simulink model "Power_System_Analysis_Protection"  (R2024b)
settings: Solver=VariableStepAuto  StartTime=0.0  StopTime=0.1  RelTol=1e-3
libraries: simulink x1, spsGroundLib x1, eePowerMeasurement x1, spsRMSLib x1, spsThreePhaseProgrammableVoltageSourceLib x1, spsThreePhaseSeriesRLCLoadLib x1, spsThreePhaseTransformerTwoWindingsLib x1, spsThreePhaseVIMeasurementLib x1, spsThreePhaseBreakerLib x1, spsThreePhaseFaultLib x1, spspowerguiLib x1
settings Model: Creator=Masoom Ali  LastModifiedBy=Masoom Ali

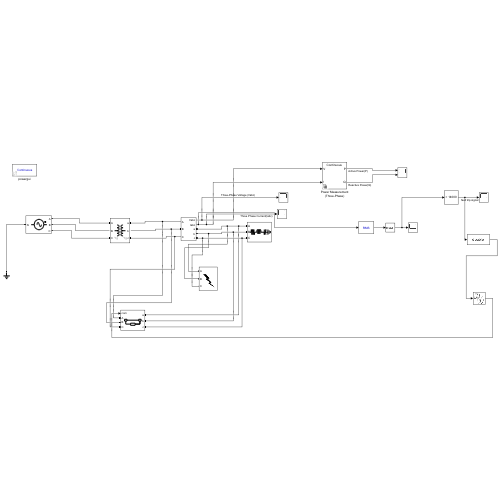
[thumbnail: Simulink's stored preview of the top-level diagram]
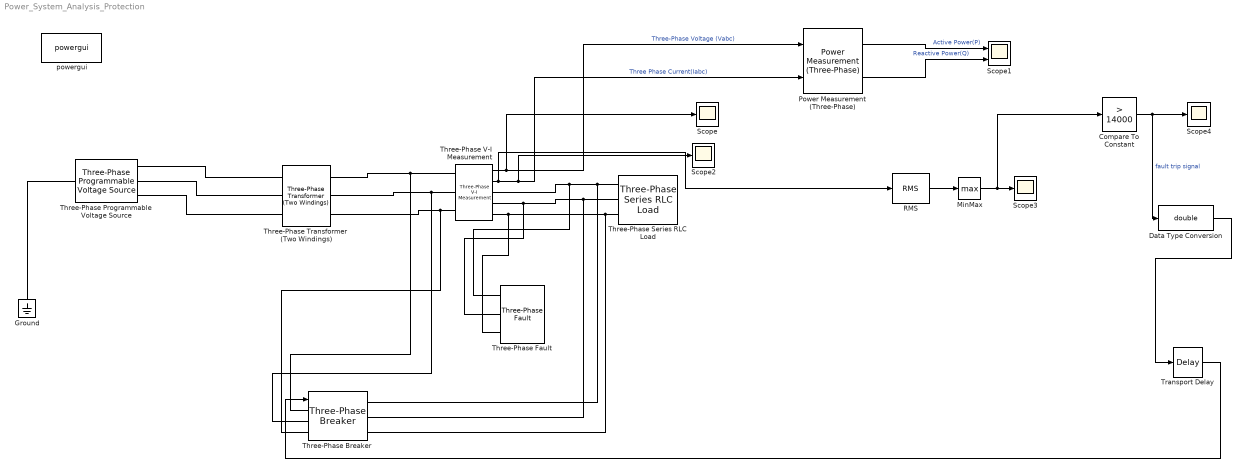
== system Power_System_Analysis_Protection ==
  Compare To Constant : simulink/Logic and Bit Operations/Compare To Constant  relop=>  const=14000  OutDataTypeStr=uint8
  Data Type Conversion : DataTypeConversion  OutDataTypeStr=double  SaturateOnIntegerOverflow=off  RndMeth=Floor
  Ground : spsGroundLib/Ground  LConnTagsString=a
  MinMax : MinMax  Function=max
  Power Measurement (Three-Phase) : eePowerMeasurement/Power Measurement (Three-Phase)  LabelModeActiveChoice=Continuous  F=50  K=1  Seq=Positive  Ts=0
  RMS : spsRMSLib/RMS  TrueRMS=on  Freq=50  RMSInit=120  Ts=0
  Scope{,2..4} (4 alike) : Scope
  Scope1 : Scope  NumInputPorts=2
  Three-Phase Programmable Voltage Source : spsThreePhaseProgrammableVoltageSourceLib/Three-Phase Programmable Voltage Source  PositiveSequence=[132e3 0 50]  VariationEntity=None  VariationType=Table of time-amplitude pairs  VariationTypeAlt=Step  VariationStep=0.5  VariationRate=10  VariationMagnitude=0.3  VariationFrequency=2  VariationTiming=[1 2]  VariationPhaseA=off  Amplitudes=[1 0.8 1.2 1.0]  TimeValues=[0 0.1 0.15 0.2]  HarmonicGeneration=off  HarmonicA=[3 0.2 -25 0]  HarmonicB=[2 0.15 35 2]  Timing="[0.05  3]"  BusType=swing  Pref=0  Qref=0  Qmin=-inf  Qmax=inf
  Three-Phase Series RLC Load : spsThreePhaseSeriesRLCLoadLib/Three-Phase Series RLC Load  LConnTagsString=A|B|C  Configuration=Y (grounded)  NominalVoltage=315e3  Vabc=[1e3 1e3 1e3]  Vabcp=[1e3 1e3 1e3]  NominalFrequency=60  UnbalancedPower=off  ActivePower=10e3  InductivePower=100  CapacitivePower=100  Pabc=[10e3 9e3 11e3]  QLabc=[100 90 110]  QCabc=[100 90 110]  Pabcp=[10e3 9e3 11e3]  QLabcp=[100 90 110]  QCabcp=[100 90 110]  Measurements=None  LoadType=constant Z
  Three-Phase Transformer (Two Windings) : spsThreePhaseTransformerTwoWindingsLib/Three-Phase Transformer (Two Windings)  Winding1Connection=Yg  Winding2Connection=Yg  CoreType=Three single-phase transformers  SetSaturation=off  Hysteresis=off  DataFile='hysteresis'  SetInitialFlux=off  Measurements=None  UNITS=pu  NominalPower=[100e6 50]  Winding1=[132e3 0.002 0.08]  Winding2=[33e3 0.002 0.08]  Rm=500  Lm=500  L0=0.5  Saturation=[ 0,0 ; 0.0024,1.2 ; 1.0,1.52 ]  InitialFluxes=[ 0.8 , -0.8 , 0.7 ]  BreakLoop=off  DiscreteSolver=Trapezoidal iterative  DataType=off  TransfoNumber=1
  Three-Phase V-I Measurement : spsThreePhaseVIMeasurementLib/Three-Phase V-I Measurement  VoltageMeasurement=phase-to-ground  SetLabelV=off  LabelV=Vabc  Vpu=off  VpuLL=off  CurrentMeasurement=yes  SetLabelI=off  LabelI=Iabc  Ipu=off  Pbase=100e6  Vbase=500e3  OutputType=Complex  PhasorSimulation=off  PSBequivalent=0
  Three-Phase Breaker : spsThreePhaseBreakerLib/Three-Phase Breaker  InitialState=closed  SwitchA=on  SwitchB=on  SwitchC=on  SwitchTimes="[1/60  5/60]"  External=on  BreakerResistance=0.01  SnubberResistance=1e6  SnubberCapacitance=inf  Measurements=None
  Three-Phase Fault : spsThreePhaseFaultLib/Three-Phase Fault  InitialStates=0  FaultA=on  FaultB=on  FaultC=on  GroundFault=on  SwitchTimes=[0.02 0.08]  External=off  SwitchStatus=NaN  FaultResistance=0.001  GroundResistance=0.01  SnubberResistance=1e6  SnubberCapacitance=inf  Measurements=Fault currents
  Transport Delay : TransportDelay
  powergui : spspowerguiLib/powergui  Priority=1  SimulationMode=Continuous  SampleTime=50e-6  frequency=60  Iterations=50  frequencyindice=50  Pbase=100e6  ErrMax=1e-4  UnitsV=kV  UnitsW=MW  buscounter=0  FunctionMessages=off  echomessages=off  EnableUseOfTLC=off  CurrentSourceSwitches=off  DisableSnubberDevices=off  DisableRonSwitches=off  DisableVfSwitches=off  DisplayEquations=off  AutomaticDiscreteSolvers=off  SolverType=Tustin/Backward Euler (TBE)  Interpol=off  ExternalGateDelay=off  methode=off  Ts=100  x0status=blocks  SPID=on  SwTol=0  HookPort=off  NonlinearTolerance=1e-4  nMaxIteration=100  ContinueOnMaxIteration=off  RestoreLinks=warning  ResistiveCurrentMeasurement=off  Frange=[0:2:500]  Ylog=off  Xlog=on  ShowGrid=off  save=off  variable=ZData  structure=0  ZoomFFT=off  StartTime=0.0  cycles=1  DisplayStyle=1  fundamental=60  FreqAxis=off  MaxFrequency=1000  frequencyindicesteady=1  RmsSteady=1  display=off
  wires:
  Power Measurement (Three-Phase)/1 -> Scope1/1  "Active Power(P)"
  Power Measurement (Three-Phase)/2 -> Scope1/2  "Reactive Power(Q)"
  Three-Phase V-I Measurement/1 -> Scope/1, Power Measurement (Three-Phase)/1  "Three-Phase Voltage (Vabc)"
  Three-Phase V-I Measurement/2 -> RMS/1, Power Measurement (Three-Phase)/2, Scope2/1  "Three Phase Current(Iabc)"
  RMS/1 -> MinMax/1
  MinMax/1 -> Compare To Constant/1, Scope3/1
  Transport Delay/1 -> Three-Phase Breaker/1
  Data Type Conversion/1 -> Transport Delay/1
  Compare To Constant/1 -> Data Type Conversion/1, Scope4/1  "fault trip signal"
  connections:
  Three-Phase Programmable Voltage Source/RConn2 -- Three-Phase Transformer (Two Windings)/LConn2
  Three-Phase Programmable Voltage Source/RConn3 -- Three-Phase Transformer (Two Windings)/LConn3
  Three-Phase Programmable Voltage Source/RConn1 -- Three-Phase Transformer (Two Windings)/LConn1
  Three-Phase V-I Measurement/LConn1 -- Three-Phase Breaker/LConn1 -- Three-Phase Transformer (Two Windings)/RConn1
  Three-Phase Transformer (Two Windings)/RConn2 -- Three-Phase Breaker/LConn2 -- Three-Phase V-I Measurement/LConn2
  Three-Phase Transformer (Two Windings)/RConn3 -- Three-Phase Breaker/LConn3 -- Three-Phase V-I Measurement/LConn3
  Three-Phase V-I Measurement/RConn2 -- Three-Phase Fault/LConn2 -- Three-Phase Breaker/RConn2 -- Three-Phase Series RLC Load/LConn2
  Three-Phase V-I Measurement/RConn3 -- Three-Phase Fault/LConn3 -- Three-Phase Breaker/RConn3 -- Three-Phase Series RLC Load/LConn3
  Ground/LConn1 -- Three-Phase Programmable Voltage Source/LConn1
  Three-Phase V-I Measurement/RConn1 -- Three-Phase Fault/LConn1 -- Three-Phase Breaker/RConn1 -- Three-Phase Series RLC Load/LConn1
